simulink model "AEB_FdFwd_Deccel"  (R2024a)
settings: Solver=FixedStepDiscrete  StartTime=0.0  StopTime=10.0  FixedStep=0.05  RelTol=1e-3
settings Model: Creator=darkh  LastModifiedBy=darkh
settings OptimizationCC: ZeroExternalMemoryAtStartup=off  ZeroInternalMemoryAtStartup=off
settings RTWCC: Description=Generate an RTMaps component embedding the model  SystemTargetFile=rtmaps.tlc  TemplateMakefile=rtmaps_default_tmf  PostCodeGenCommand=rtmaps_post_code_generation(buildInfo)  RetainRTWFile=on  TargetLang=C++
settings STFCustomTargetCC: TargetLangStandard=C++11 (ISO)  ModelReferenceCompliant=off  ConcurrentExecutionCompliant=on  CombineOutputUpdateFcns=on  CodeInterfacePackaging=C++ class  CPPClassGenCompliant=on  GRTInterface=off  UseToolchainInfoCompliant=off  SystemTargetFile=rtmaps.tlc
settings GRTTargetCC: TargetLangStandard=C++11 (ISO)  ModelReferenceCompliant=off  ParMdlRefBuildCompliant=off  CompOptLevelCompliant=off  MatFileLogging=off  CodeInterfacePackaging=C++ class  UseToolchainInfoCompliant=off

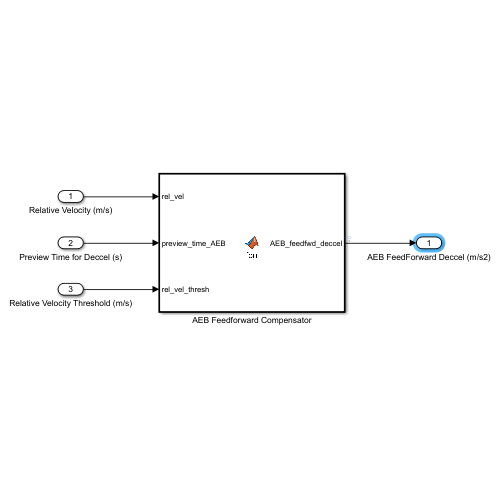
[thumbnail: Simulink's stored preview of the top-level diagram]
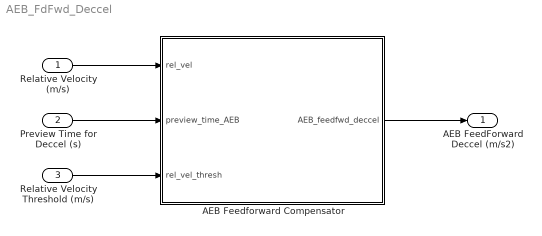
== system AEB_FdFwd_Deccel ==
  Relative Velocity (m/s) : Inport
  Preview Time for Deccel (s) : Inport  Port=2
  Relative Velocity Threshold (m/s) : Inport  Port=3
  AEB Feedforward Compensator : MATLAB Function  TreatAsAtomicUnit=on
  AEB FeedForward Deccel (m/s2) : Outport
  wires:
  Relative Velocity (m/s)/1 -> AEB Feedforward Compensator/1(rel_vel)
  Preview Time for Deccel (s)/1 -> AEB Feedforward Compensator/2(preview_time_AEB)
  Relative Velocity Threshold (m/s)/1 -> AEB Feedforward Compensator/3(rel_vel_thresh)
  AEB Feedforward Compensator/1(AEB_feedfwd_deccel) -> AEB FeedForward Deccel (m/s2)/1

== matlab function AEB_FdFwd_Deccel/AEB Feedforward Compensator ==
  data: rel_vel input; AEB_feedfwd_deccel output; preview_time_AEB input; rel_vel_thresh input
function AEB_feedfwd_deccel = fcn(rel_vel, preview_time_AEB, rel_vel_thresh)
% This function determines a feedforward decceleration to apply to vehicle
% in the event that the vehicle approaches a stopped car at high speed,
% i.e. Automatic Emergency Braking (AEB) event
% rel_vel is the relative velocity compared to lead vehicle [m/s]; 
% preview_time is the time in [secs] over which the car should slow down based on the relative velocity; 
% rel_vel_thresh is the relative velocity threshold, smaller relative velocity differences than this value will be ignored [m/s]

if rel_vel > -rel_vel_thresh
    AEB_feedfwd_deccel = 0.0;
    return;
end

AEB_feedfwd_deccel = rel_vel/preview_time_AEB;
